simulink model "multichannel_creater"  (R2017b)
settings: Solver=FixedStepDiscrete  StartTime=0.0  StopTime=60  RelTol=1e-3  EnableMultiTasking=on
model workspace (MAT data in the model file):
  MCOS : class17 (value not decoded)
  heli = [0 -3.0517578125e-05 -0.0001220703125 -0.000244140625 -0.0003662109375 -0.000701904296875 -0.00106811523438 -0.00204467773438 -0.00341796875 -0.00460815429688 -0.00595092773438 -0.00762939453125 ... (263304 elements, 263304x1)]
libraries: dspvision x4, dspindex x2
(part 2 of 2)

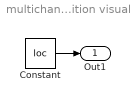
== system multichannel_creater/ Set position visually ==
  Constant : Constant  Value=loc  VectorParams1D=off  SampleTime=-1
  Out1 : Outport
  wires:
  Constant/1 -> Out1/1

== matlab function multichannel_creater/Set position randomly ==
  data: loc output
function loc = randomLoc()
% This block Computes a random position in a unit circle. 

persistent lastLoc;

if isempty(lastLoc)
    lastLoc = [0 0.5];
end

lastLoc = lastLoc + 0.02*randn(1,2);
nrm = norm(lastLoc);
if nrm > 1
    lastLoc = lastLoc / nrm;
end
loc = lastLoc;

== matlab function multichannel_creater/Speaker volume computation ==
  data: pos input; mix output
function mix = computeVol(pos)
% This block Computes a speaker mixing matrix based on
% the source location. 

% left front
% right front
% front center
% low frequency
% left rear
% right rear

% x,y speaker locations
speakerLoc = [-1 1; 1 1; 0 sqrt(2); -1 -1; 1 -1] ./ sqrt(2);

sourceDistance = norm(pos);
sourceDir      = pos / sourceDistance;

amp = 0.5 * (speakerLoc * pos');
[dist, ndx] = sort(amp, 'descend');
sideMix = [0 0 0 0 0];

% Determine the vector of speaker amplitudes
if sourceDistance == 0
    % They are dead center.
% Can we represent the sound with one speaker?
elseif dist(1) == sourceDistance
    sideMix(ndx(1)) = 1;
    
% OK, split the sound between speakers.
else
    % Find the closest vector.
    closest = ndx(1:2);
    % The second 'closest' vector is the closest vector to the source 
    % which is further away from the closest vector.
    for i=2:length(ndx)
        if speakerLoc(closest(1),:) * speakerLoc(ndx(i),:)' > ...
           sourceDir * speakerLoc(ndx(i),:)'
           closest(2) = ndx(i+1);
        else
            break;
        end
    end
    % Express the source direction using the nearest two speaker vectors
    % as a basis
    p = sourceDir;
    L = speakerLoc(closest, :);
    g = p/L;
    % Re-normalize.
    % This is really only necessary for the center channel.
    g = g/norm(g);
    sideMix(closest) = g;
end


% We computed the balance as if the source were on the unit circle.
% In the middle of the cirle, this algorithm will produce an effect 
% which is too "discrete".  Hence, we will cross-fade to the outer ring 
% from a center where we assume that all speakers are on.
 

% Set all speaker amplitudes equal when in the center.
centerMix = ones([1 6]);

% Mix from the center to the side allocation strategy, and then normalize 
% the power so that it remains constant.
centerFalloff = (1-sourceDistance)^2;
mix = centerMix*centerFalloff +...
    + [sideMix(1:3) 0 sideMix(4:5)]*(1-centerFalloff);
mix = mix / norm(mix);

% Finally, adjust the amplitude so that it falls off with an inverse 
% square law, and the perimeter is 1/4 as loud as the center.  Since we 
% know that the maximum amplitude of a channel is 1/sqrt(6) (which happens 
% in the center), we multiply by sqrt(6). 
mix = sqrt(6) * mix * (1/(1+sourceDistance))^2;
end
